simulink model "twotimes3003"  (R2018b)
settings: Solver=VariableStepAuto  StartTime=0.0  StopTime=10.0  RelTol=1e-3
settings Model: Creator=student  LastModifiedBy=student

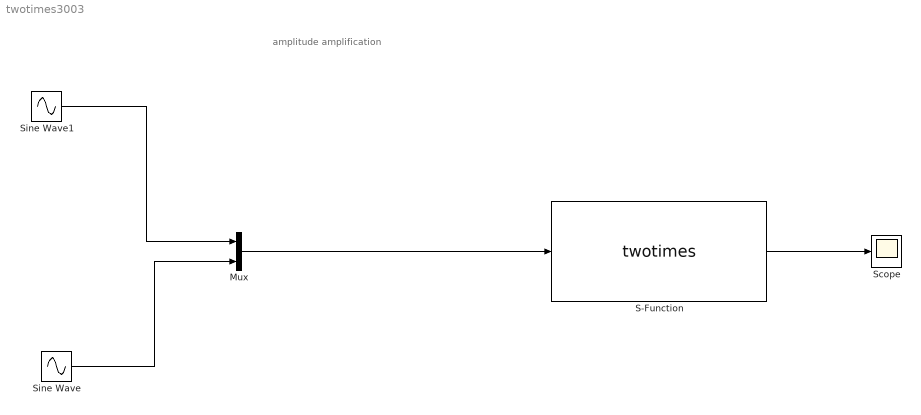
== system twotimes3003 ==
  note: amplitude amplification
  Mux : Mux  Inputs=2
  S-Function : S-Function  FunctionName=twotimes  Parameters=5  SFunctionDeploymentMode=off  EnableBusSupport=off
  Scope : Scope
  Sine Wave : Sin  SampleTime=0
  Sine Wave1 : Sin  Amplitude=2  SampleTime=0
  wires:
  S-Function/1 -> Scope/1
  Sine Wave1/1 -> Mux/1
  Sine Wave/1 -> Mux/2
  Mux/1 -> S-Function/1
